simulink model "main"  (R2025b)
settings: Solver=VariableStepAuto  StartTime=0.0  StopTime=10  FixedStep=0.01  RelTol=1e-3
values from neighbouring files (symbols this model uses):
  dist = [100, 100, -50]    [skrypt.m]
  fs = 100    [skrypt.m]
  v_obejcts = [20 40 40]    [skrypt.m]
  y_pos = [2 3 6]    [skrypt.m]
libraries: simulink x2
settings Model: Creator=julia  LastModifiedBy=julia

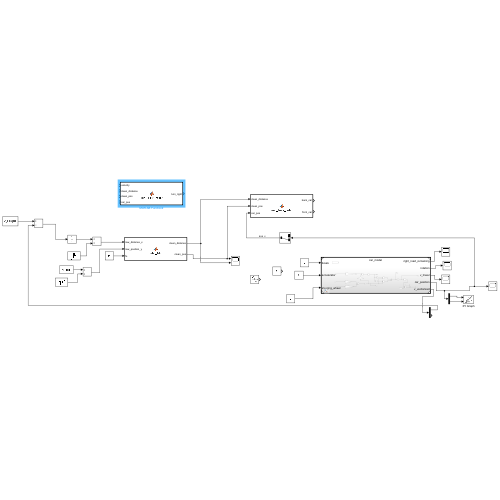
[thumbnail: Simulink's stored preview of the top-level diagram]
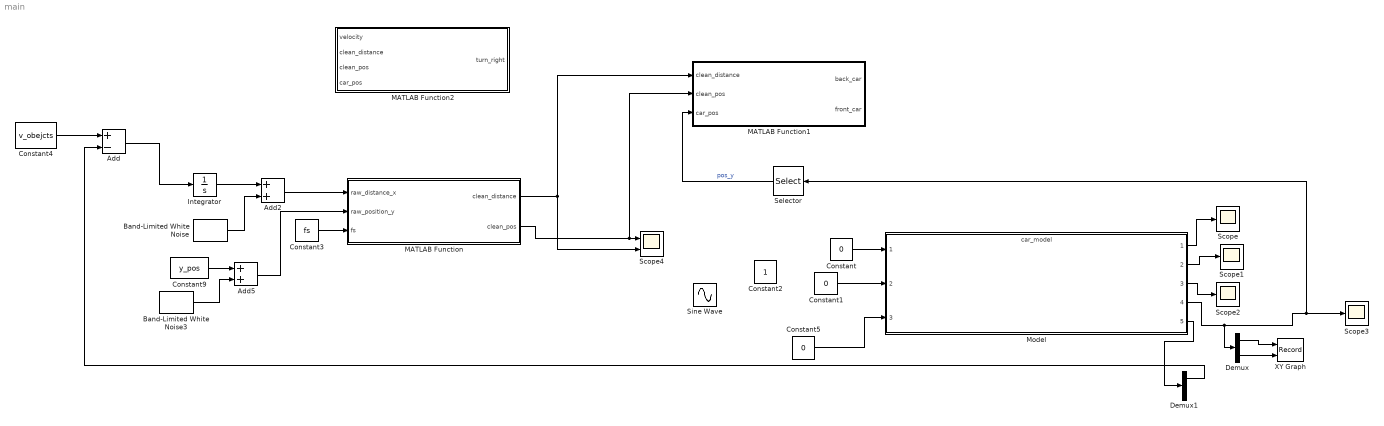
== system main ==
  Add : Sum  Inputs=+-
  Add2 : Sum
  Add5 : Sum
  Band-Limited White Noise : simulink/Sources/Band-Limited White Noise  Cov=[0.1]  Ts=0.1  seed=[23341]
  Band-Limited White Noise3 : simulink/Sources/Band-Limited White Noise  Cov=[0.1]  Ts=0.1  seed=[23341]
  Constant : Constant  Value=0
  Constant1 : Constant  Value=0
  Constant2 : Constant
  Constant3 : Constant  Value=fs
  Constant4 : Constant  Value=v_obejcts
  Constant5 : Constant  Value=0
  Constant9 : Constant  Value=y_pos
  Demux : Demux  Outputs=2
  Demux1 : Demux  Outputs=2
  Integrator : Integrator  InitialCondition=dist
  MATLAB Function : MATLAB Function  TreatAsAtomicUnit=on
  MATLAB Function1 : MATLAB Function  TreatAsAtomicUnit=on
  MATLAB Function2 : MATLAB Function  TreatAsAtomicUnit=on
  Model : ModelReference  ModelNameDialog=car_model.slx  SimulationMode=Normal  ModelReferenceVersion=1.3
  Scope{,1..3} (4 alike) : Scope
      Scope1 settings: ActiveDisplayYMinimum=-1  ActiveDisplayYMaximum=1
      Scope2 settings: DataLoggingVariableName=ScopeData2
      Scope3 settings: ActiveDisplayYMinimum=-145.41907628081782  ActiveDisplayYMaximum=403.34212677962563  DataLoggingVariableName=ScopeData3
  Scope4 : Scope  NumInputPorts=2
      settings: ActiveDisplayYMinimum=-191.9275934660821  ActiveDisplayYMaximum=339.07595938553436  DataLoggingVariableName=ScopeData4
  Selector : Selector  InputPortWidth=2  IndexOptions=Index vector (dialog)  Indices=[2]  OutputSizes=1
  Sine Wave : Sin  Amplitude=0.5  SampleTime=0
  XY Graph : Record  NumPorts=2.0  FileSettingsInternal="{\"entries\":[{\"content\":{\"excelSettings\":{\"content\":{},\"type\":\"Streamout.ExcelSettings\"},\"parquetSettings\":{\"content\":{},\"type\":\"Streamout.ParquetSettings\"}},\"type\":\"Streamout.FileSettingStorage\",\"uuid\":\"\"}],\"packageUris\":[\"http:\\/\\/schema.mathworks.com\\/mf0\\/streamout_blocks\\/R2020a\"],\"version\":\"1.0\"}"  FrameSettings=[0, 0]  Layout=[1 1]  SignalsInternal="{\"entries\":[{\"content\":{\"signals\":[{\"content\":{\"blockPath\":[],\"dimensions\":[1],\"domain\":\"\",\"lineColor\":\"#a2142f\",\"plots\":[ 1 ],\"port\":1,\"sid\":[\"\"],\"signalID\":1,\"signalName\":\"Demux:1\"},\"type\":\"RecordBlkView.Signal\",\"uuid\":\"\"},{\"content\":{\"blockPath\":[],\"dimensions\":[1],\"domain\":\"\",\"lineColor\":\"#139fff\",\"plots\":[ 1 ],\"port\":2,\"sid\":[\"\"],\"signalID\":2,\"signalName\":\"Demux:2\"},\"type\":\"RecordBlkView.Signal\",\"uuid\":\"\"}]},\"type\":\"RecordBlkView.InputSignals\",\"uuid\":\"\"}],\"packageUris\":[\"http:\\/\\/schema.mathworks.com\\/mf0\\/streamout_blocks\\/R2020a\"],\"version\":\"1.0\"}"  VisualizationBindings="{\"xyplotplugin\":{\"info\":[{\"series\":[{\"bindingParametersList\":[{\"parameter\":\"X-Axis\",\"signalID\":1,\"signalName\":\"Demux:1\"},{\"parameter\":\"Y-Axis\",\"signalID\":2,\"signalName\":\"Demux:2\"}],\"seriesID\":0}],\"subplotID\":1}]}}"  CompatibilityTag=XY
  wires:
  Constant/1 -> Model/1
  Model/1 -> Scope/1
  Model/2 -> Scope1/1
  Model/3 -> Scope2/1
  Model/4 -> Demux/1, Selector/1, Scope3/1
  Demux/1 -> XY Graph/1
  Demux/2 -> XY Graph/2
  Constant3/1 -> MATLAB Function/3(fs)
  Band-Limited White Noise/1 -> Add2/2
  Add2/1 -> MATLAB Function/1(raw_distance_x)
  Integrator/1 -> Add2/1
  MATLAB Function/1(clean_distance) -> MATLAB Function1/1(clean_distance), Scope4/2
  Constant4/1 -> Add/1
  Add/1 -> Integrator/1
  Model/5 -> Demux1/1
  Demux1/1 -> Add/2
  Constant5/1 -> Model/3
  Band-Limited White Noise3/1 -> Add5/2
  Constant9/1 -> Add5/1
  Add5/1 -> MATLAB Function/2(raw_position_y)
  MATLAB Function/2(clean_pos) -> MATLAB Function1/2(clean_pos), Scope4/1
  Constant1/1 -> Model/2
  Selector/1 -> MATLAB Function1/3(car_pos)  "pos_y"

== matlab function main/MATLAB Function1 ==
  settings: updateMethod=DISCRETE
  data: clean_distance input; clean_pos input; back_car output; front_car output; car_pos input
function [back_car, front_car] = front_back_radar(clean_distance, clean_pos, car_pos)

in_line_distance = [];
for i = 1:length(clean_distance)
    if clean_pos(i) > car_pos - 1 && clean_pos < car_pos + 1
        in_line_distance(end+1) = clean_distance(i);
    end
end
    

front = in_line_distance(in_line_distance > 0);
back = in_line_distance(in_line_distance < 0);

if ~isempty(front)
    front_car = min(front);
else
    front_car = NaN;
end

if ~isempty(back)
    back_car = max(back);
else
    back_car = NaN;
end
end

== matlab function main/MATLAB Function ==
  settings: updateMethod=DISCRETE
  data: raw_distance_x input; raw_position_y input; clean_distance output; fs input; clean_pos output
function [clean_distance, clean_pos] = radar_filter(raw_distance_x, raw_position_y, fs)
    persistent last_dist;
    persistent last_pos;
    
    n_objects = length(raw_distance_x);
    
    dt    = 1 / fs;
    tau   = 0.02;
    alpha = dt / (tau + dt);

    % isempty() MUSI być sprawdzone jako pierwsze i osobno
    if isempty(last_dist)
        last_dist = raw_distance_x;
        last_pos  = raw_position_y;
    end

    % Dopiero TU (po przypisaniu) można używać length/size
    if length(last_dist) ~= n_objects
        last_dist = raw_distance_x;
        last_pos  = raw_position_y;
    end

    clean_distance = alpha * raw_distance_x + (1 - alpha) * last_dist;
    clean_pos      = alpha * raw_position_y  + (1 - alpha) * last_pos;
    
    last_dist = clean_distance;
    last_pos  = clean_pos;
end

== matlab function main/MATLAB Function2 ==
  settings: updateMethod=DISCRETE
  data: velocity input; clean_distance input; clean_pos input; turn_right output; car_pos input
function turn_right  = front_back_radar(velocity, clean_distance, clean_pos, car_pos)

right_car_dist = [];
right_car_vel = [];
for i = 1:length(clean_distance)
    if clean_pos(i) > car_pos + 2 && clean_pos < car_pos + 5
        right_car_dist(end+1) = clean_distance(i);
        right_car_vel(end+1) = velocity(i);
    end
end

if all(right_car_vel .* 5 < (right_car_dist - 1))
    turn_right = true;
else
    turn_right = false;
end
end
